simulink model "Dc_motor_assignment"  (R2023a)
settings: Solver=VariableStepAuto  StartTime=0.0  StopTime=3  RelTol=1e-3
values from neighbouring files (symbols this model uses):
  B = 0.1    [Dc_ASSIGNMENT_INPUTS.m]
  J = 0.01    [Dc_ASSIGNMENT_INPUTS.m]
  L = 0.5    [Dc_ASSIGNMENT_INPUTS.m]
settings Model: LastModifiedBy=mluser

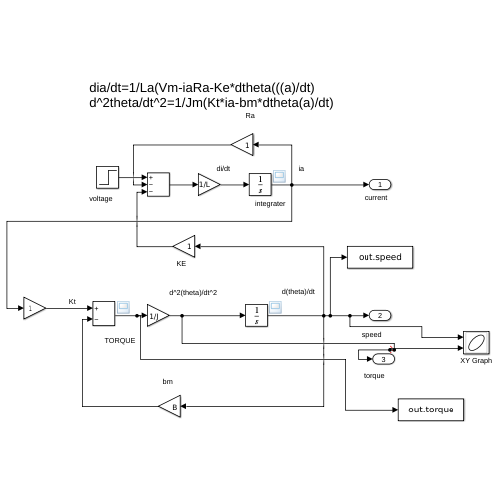
[thumbnail: Simulink's stored preview of the top-level diagram]
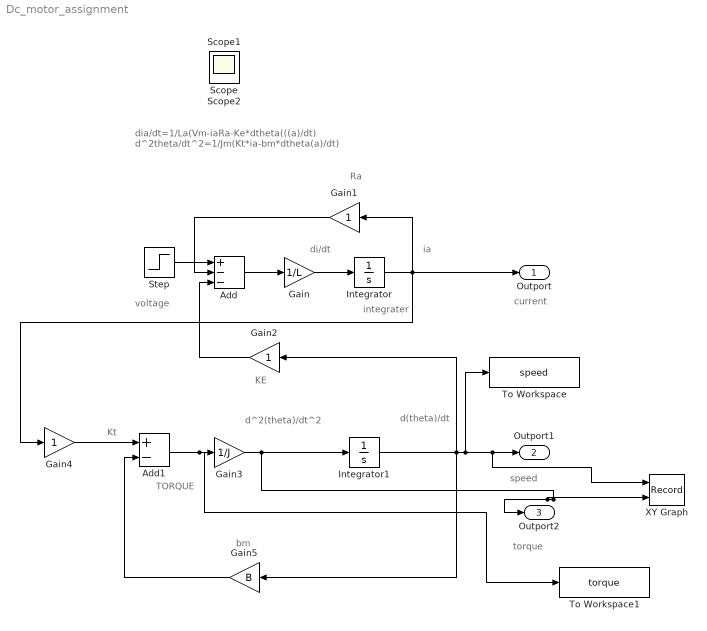
== system Dc_motor_assignment ==
  note: bm
  note: torque
  note: speed
  note: current
  note: Ra
  note: ia
  note: di/dt
  note: TORQUE
  note: KE
  note: Kt
  note: d(theta)/dt
  note: d^2(theta)/dt^2
  note: integrater
  note: voltage
  note: dia/dt=1/La(Vm-iaRa-Ke*dtheta(((a)/dt)
      | d^2theta/dt^2=1/Jm(Kt*ia-bm*dtheta(a)/dt)
  Add : Sum  Inputs=+--
  Add1 : Sum  Inputs=+-
  Gain : Gain  Gain=1/L
  Gain1 : Gain
  Gain2 : Gain
  Gain3 : Gain  Gain=1/J
  Gain4 : Gain
  Gain5 : Gain  Gain=B
  Integrator : Integrator
  Integrator1 : Integrator
  Step : Step  After=230  SampleTime=0
  To Workspace : ToWorkspace  VariableName=speed  SaveFormat=Timeseries  SampleTime=-1
  To Workspace1 : ToWorkspace  VariableName=torque  SaveFormat=Timeseries  SampleTime=-1
  XY Graph : Record  FileSettingsInternal="{\"entries\":[{\"content\":{\"excelSettings\":{\"content\":{},\"type\":\"Streamout.ExcelSettings\"}},\"type\":\"Streamout.FileSettingStorage\",\"uuid\":\"\"}],\"packageUris\":[\"http:\\/\\/schema.mathworks.com\\/mf0\\/streamout_blocks\\/R2020a\"],\"version\":\"1.0\"}"  Layout=[1 1]  SignalsInternal="{\"entries\":[{\"content\":{\"signals\":[{\"content\":{\"blockPath\":[],\"dimensions\":[1],\"domain\":\"\",\"lineColor\":\"#a2142f\",\"plots\":[1],\"port\":1,\"sid\":[\"\"],\"signalID\":206,\"signalName\":\"Integrator1\"},\"type\":\"RecordBlkView.Signal\",\"uuid\":\"\"},{\"content\":{\"blockPath\":[],\"dimensions\":[1],\"domain\":\"\",\"lineColor\":\"#139fff\",\"plots\":[1],\"port\":2,\"sid\":[\"\"],\"signalID\":210,\"signalName\":\"Gain3\"},\"type\":\"RecordBlkView.Signal\",\"uuid\":\"\"}]},\"type\":\"RecordBlkView.InputSignals\",\"uuid\":\"\"}],\"packageUris\":[\"http:\\/\\/schema.mathworks.com\\/mf0\\/streamout_blocks\\/R2020a\"],\"version\":\"1.0\"}"  VisualizationBindings="{\"xyplotplugin\":{\"info\":[{\"series\":[{\"bindingParametersList\":[{\"parameter\":\"X-Axis\",\"signalID\":206,\"signalName\":\"Integrator1\"},{\"parameter\":\"Y-Axis\",\"signalID\":210,\"signalName\":\"Gain3\"}],\"seriesID\":30853}],\"subplotID\":1}]}}"  CompatibilityTag=XY
  Outport : Outport
  Outport1 : Outport  Port=2
  Outport2 : Outport  Port=3
  Scope : Scope
  Scope1 : Scope
  Scope2 : Scope
  wires:
  Step/1 -> Add/1
  Add/1 -> Gain/1
  Gain/1 -> Integrator/1
  Integrator/1 -> Gain4/1, Gain1/1, Outport/1
  Gain1/1 -> Add/2
  Gain2/1 -> Add/3
  Integrator1/1 -> Gain5/1, Gain2/1, XY Graph/1, Outport1/1, To Workspace/1
  Gain3/1 -> XY Graph/2, Outport2/1, Integrator1/1
  Gain4/1 -> Add1/1
  Add1/1 -> To Workspace1/1, Gain3/1
  Gain5/1 -> Add1/2
